simulink model "tank_no_controller"  (R2013a)
settings: Solver=ode45  StartTime=0.0  StopTime=100  RelTol=1e-3
undefined symbols (not defined in the file): A, kv, R
libraries: simulink x1
settings Model: Creator=Ahmed  LastModifiedBy=Ahmed

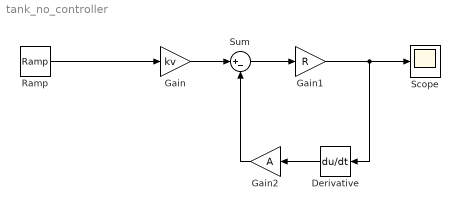
== system tank_no_controller ==
  Derivative : Derivative
  Gain : Gain  Gain=kv
  Gain1 : Gain  Gain=R
  Gain2 : Gain  Gain=A
  Ramp : simulink/Sources/Ramp  slope=1  start=0  X0=0
  Scope : Scope
  Sum : Sum  Inputs=|+-
  wires:
  Gain/1 -> Sum/1
  Ramp/1 -> Gain/1
  Sum/1 -> Gain1/1
  Gain1/1 -> Derivative/1, Scope/1
  Derivative/1 -> Gain2/1
  Gain2/1 -> Sum/2
